simulink model "OscillatorAndLockin_Phase_or_Amp_FB_Mode"  (R2022b)
settings: Solver=VariableStepAuto  StartTime=0.0  StopTime=0.1  RelTol=1e-3
model workspace: external: MAT-File C:\Users\yoni\Documents\MATLAB\Examples\AFM\Dynamic Mode\WorkSpaceData.mat (data not in the file)
undefined symbols (not defined in the file or in its folder): ClockPeriod, D, I, N, P
libraries: simulink x7, slpidlib x2, simulink_extras x1
Description:
  | A model of the workings of "Phase or Amplitude feedback AFM (Atomic Force Microscopy)" aka "Tapping mode AFM"
  | This model contains:
  | a model of an AFM tip made of a tuning fork with tip-sample interaction force  i.e. a damped harmonic oscillator with external forces applied.
  | a model of a "Lock-in Amplifier",  with PLL mechanism that tracks the oscillator frequency.
  | 
  | The lock-in Amplifier does a "convolution" by multiplying its internal reference sin and cos signals with oscillator position signal, and summing each tick within a "time constant" period.
  | This splits the signal into symetric (cos) and antisymetric (sin) components. using euler
  | θ = tan-1 ( y / x )     r = √ ( x2 + y2 )
  | we can get esteemates for theta (phase) and r (amplitude)
  | lock-in then sythesize a sin signal amplitude of 1 and +90 degrees phase from the original position.
  | The oscillator is driven at it's own resonance frequency with a constant amplitude.
  | This is done by a controlled positive feedback loop, Autoresonance's force is amplified by a value designed to keep amplitude constant at setpoint.
  | (using a PID and the Lock-in's amplitude estimation)
  | 
  | The lock-in and PLL model uses the lock-in calculated phase and use that value to correct the lock-in's internal frequency
  | so it will match the external oscillator's frequency. (using another PID)
settings Model: PacingRate=1000  VariantFading=off  Creator=Yoni Cohen  LastModifiedBy=yoni
settings ConfigSet: Description=Current Conf
settings SolverCC: ZeroCrossAlgorithm=Adaptive  AlgebraicLoopSolver=LineSearch
settings DebuggingCC: UnconnectedInputMsg=warning  UnconnectedOutputMsg=warning  UnconnectedLineMsg=warning  UniqueDataStoreMsg=error  SFMachineParentedDataDiag=warning
settings HardwareCC: TargetBitPerPointer=64  TargetBitPerSizeT=64  TargetBitPerPtrDiffT=64  TargetLargestAtomicFloat=Float  TargetIntDivRoundTo=Zero  TargetEndianess=LittleEndian  TargetWordSize=64  TargetHWDeviceType=Intel->x86-64 (Windows64)  ProdEqTarget=off
settings ModelReferenceCC: EnableRefExpFcnMdlSchedulingChecks=on
settings SFSimCC: CustomCodeUndefinedFunction=UseInterfaceOnly

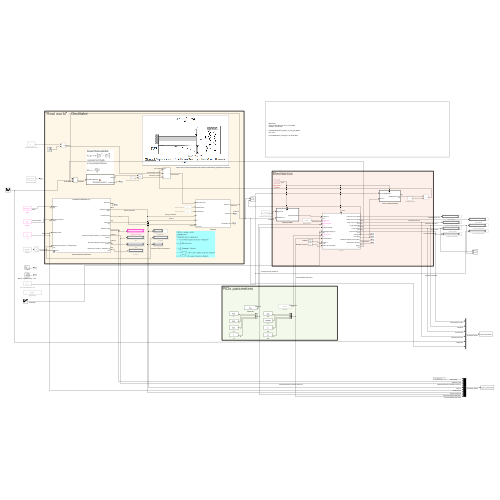
[thumbnail: Simulink's stored preview of the top-level diagram]
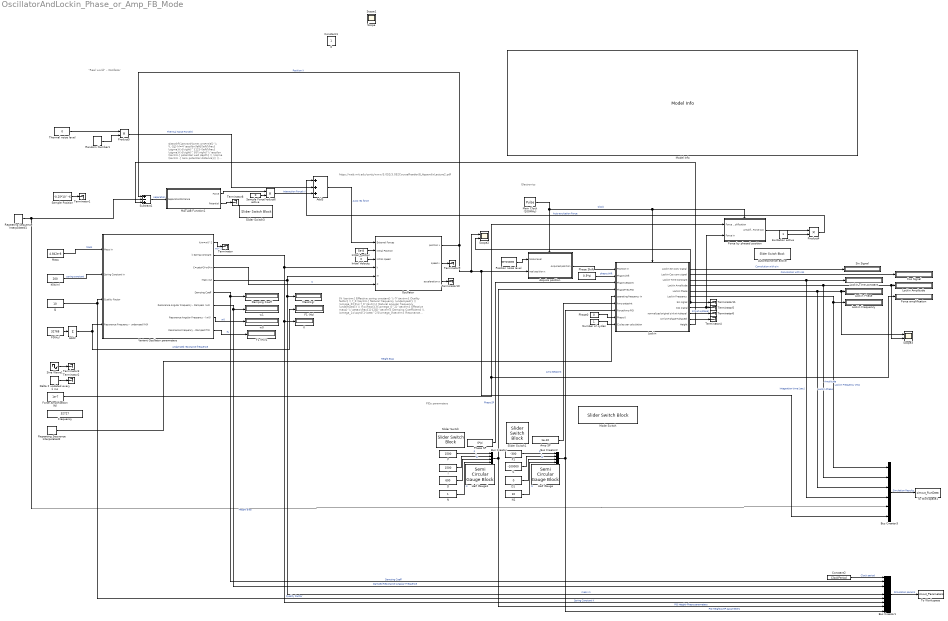
== system OscillatorAndLockin_Phase_or_Amp_FB_Mode ==
  note: $\textbf{Lennard-Jones potential} \\ V_{LJ}(r)=4 \epsilon\left[\left(\frac{ \sigma}{r}\right)^{12}-\left(\frac{ \sigma}{r}\right)^{6}\right] \\ \epsilon \textrm{ potential well depth} \\ \sigma \textrm { zero potential distance}\\ \\ F(r)=-\frac{\mathrm{d}V(r)}{\mathrm{d}r}$
  note: https://web.mit.edu/cortiz/www/3.052/3.052CourseReader/8_AppendixLecture2.pdf
  note: "Real world" - Oscillator
  note: Electronics
  note: PIDs parameters
  note: $k \textrm{ Effective spring constant} \\ Q \textrm{ Quality factor} \\ f_0 \textrm{ Natural frequency (undamped)} \\ \omega_0=2\pi f_0 \textrm{ Natural angular frequency (undamped)} \\ m=\frac{k}{\omega_0^2} \textrm{ Effective mass} \\ \zeta=\frac{1}{2Q} \textrm{ Damping Coefficient} \\ \omega_1=\sqrt{(1-\zeta^2)}\omega_0\textrm{ Resonance angular frequency (damped)} \\ f_1= \sqrt{(1-\zeta^2)}f_0\textrm{ Resonance frequency (damped)}$
  Acquire position : Subsystem
  Add2 : Sum  Inputs=+
  Add3 : Sum  Inputs=+++
  Amp SP : Constant  Value=1e-10  VectorParams1D=off  SampleTime=1e-5
  Autoresonance active : SliderSwitchBlock
      settings: Values={{'Off', 'On'}, [0 1]}
  Bus Creator : BusCreator  Inputs=P,I,D,N
  Bus Creator1 : BusCreator  Inputs=9
  Bus Creator2 : BusCreator  Inputs=P,I,D,N
  Bus Creator3 : BusCreator  Inputs=6
  Constant2 : Constant  Value=ClockPeriod
  Cos Signal : Display
  D : Constant  Value=600  SampleTime=1e-5
  D1 : Constant  Value=0  SampleTime=1e-5
  Damping Coeff : Display
  Delta F updated every 1 ms : RandomNumber  Variance=100  Seed=7546745  SampleTime=1e-3
  Excitation active : Constant  SampleTime=-1
  F0(Hz) : Constant  Value=32768
  F1 (Hz) : Display
  F1 (Hz)1 : Display
  Force Amplification (N) : Constant  Value=1e-7  SampleTime=-1
  Force amplification : Display
  Force by phased position : Subsystem  VariantControl=true
  Frequency : Constant  Value=32727  SampleTime=-1
  Half Gauge : SemiCircularGaugeBlock  LabelPosition=Bottom  ScaleMin=-10e-11  ScaleMax=10e-11
  Half Gauge1 : SemiCircularGaugeBlock  LabelPosition=Bottom  ScaleMin=-5e-4  ScaleMax=5e-4
  I : Constant  Value=1500  SampleTime=1e-5
  I1 : Constant  Value=-100000  VectorParams1D=off  SampleTime=1e-5
  Initial Position : Constant  Value=5e-8  VectorParams1D=off
  Initial Velocity : Constant  Value=0
  K : Display
  K(N/m) : Constant  Value=200
  Lockin : Subsystem
  Lockin Amplitude : Display
  Lockin Frequency : Display
  Lockin Phase : Display
  Lockin Time constant : Display
  MATLAB Function1 : MATLAB Function  TreatAsAtomicUnit=on
  Main Clock (100MHz) : DiscretePulseGenerator  PulseType=Time based  Period=ClockPeriod  PulseWidth=50
  Mass : Constant  Value=4.842e-8
  Mass(kg) : Display
      settings: Format=short_e
  Mode Switch : SliderSwitchBlock
      settings: Values={{'Amplitude FB', 'Phase FB'}, [0 1]}
  Model Info : simulink/Model-Wide Utilities/Model Info  Frame=on  DisplayStringWithTags=|  HorizontalTextAlignment=Left  LeftAlignmentValue=0.02
      | Model Info
      | Date Created %<Created>
      | Creator : %<Creator>
      | %<ModifiedComment>
      | %<ModelName> 
      | Ver. %<ModelVersion>
      | %<Description>
      | Last modification: %<LastModificationDate>
  N : Constant  SampleTime=1e-5
  N1 : Constant  Value=10  SampleTime=1e-5
  Number of cycles : Constant  OutDataTypeStr=uint16  SampleTime=-1
  Oscillator : Subsystem
  P : Constant  Value=1500  SampleTime=1e-5
  P1 : Constant  Value=-300  SampleTime=1e-5
  Phase SP : Constant  Value=0*pi  SampleTime=1e-5
  Phase Shift : Constant  Value=0.5*pi  VectorParams1D=off  SampleTime=-1
  Phase0 : Constant  Value=0  SampleTime=-1
  Position noise level : Constant  Value=0e-9/10000  VectorParams1D=off  SampleTime=-1
  Product4 : Product
  Product5 : Product
  Product6 : Product
  Q : Constant  Value=10
  Random Number1 : RandomNumber  Seed=754666  SampleTime=10^-8
  Repeating Sequence Interpolated1 : simulink/Sources/Repeating Sequence Interpolated  OutValues="[25e-10  0.6e-9 25e-10]"  TimeValues=[0 0.3 0.6]  LookUpMeth=Interpolation-Use End Values  tsamp=10^-5  OutMin=[]  OutMax=[]  OutDataTypeStr=double  OutputDataTypeScalingMode=double  OutDataType=fixdt(0,8)  OutScaling=2^-10
  Repeating Sequence Interpolated2 : simulink/Sources/Repeating Sequence Interpolated  OutValues="[32720  32800 32800]"  TimeValues=[0 0.1 0.11]  LookUpMeth=Interpolation-Use End Values  tsamp=10^-5  OutMin=[]  OutMax=[]  OutDataTypeStr=double  OutputDataTypeScalingMode=double  OutDataType=fixdt(0,8)  OutScaling=2^-10
  Sample Force active : Constant  Value=0  SampleTime=-1
  Sample Position : Constant  Value=-0.25*10^-6  SampleTime=-1
  Scope2 : Scope  NumInputPorts=2
  Scope3 : Scope  NumInputPorts=2
  Sin Signal : Display
  Sine Wave1 : Sin  Amplitude=20  Frequency=5000  Phase=0.0001  SampleTime=10e-6
  Slider Switch : SliderSwitchBlock
      settings: Values={{'Off', 'On'}, [0 1]}
  Slider Switch1 : SliderSwitchBlock
      settings: Values={{'Off', 'On'}, [0 1]}
  Slider Switch3 : SliderSwitchBlock
      settings: Values={{'Off', 'On'}, [0 1]}
  Subtract1 : Sum  Inputs=+-+  OutMin=[0]  RndMeth=Nearest
  Terminator{,1..6,8..11} (11 alike) : Terminator
  Thermal noise level : Constant  Value=0  VectorParams1D=off  SampleTime=-1
  To Workspace : ToWorkspace  VariableName=simout_Parameters  SaveFormat=Timeseries  SampleTime=1
  To Workspace1 : ToWorkspace  VariableName=simout_RunData  SaveFormat=Timeseries  SampleTime=1e-5
  Variant Oscillator parameters : Subsystem  Description=|  Variant=on  VariantControlMode=label  LabelModeActiveChoice=OscillatorTypeVar==0  PropagateVariantConditions=on
      | k  \textrm{ Effective spring constant.}
      | \\
      | Q  \textrm{ Quality factor.}
      | \\
      | f_0  \textrm{ Natural frequency undamped.}
      | \\
      | \omega_0=2\pi f_0 \textrm{ Natural angular frequency.}
      | \\
      | m=\frac{k}{\omega_0^2}  \textrm{ Effective mass.}
      | \\
      | \zeta=\frac{1}{2Q} \textrm{ Damping Coefficient.}
      | \\
      | \omega_1=\sqrt{(1-\zeta^2)}\omega_0\textrm{ Resonance angular frequency (damped)}
      | \\
      | f_1= \omega_1=\sqrt{(1-\zeta^2)}f_0\textrm{ Resonance frequency (damped)}
  w0 : Display
  w1 : Display
  0 : Constant  IOType=siggen
  Constant1 : Constant  IOType=siggen
  Scope : Scope
  Scope1 : Scope
  wires:
  Main Clock (100MHz)/1 -> Lockin/Trigger, Force by phased position/Trigger, Acquire position/Trigger  "Clock"
  Force by phased position/1(Amplified Force out) -> Product4/1
  Phase Shift/1 -> Lockin/2(Phase shift)  "phase shift"
  F0(Hz)/1 -> Add2/1
  Excitation active/1 -> Product4/2
  Random Number1/1 -> Product5/2
  Thermal noise level/1 -> Product5/1
  Sample Force active/1 -> Product6/2
  MATLAB Function1/1(Force) -> Product6/1
  Subtract1/1 -> MATLAB Function1/1(SeparationDistance)  "separation"
  K(N/m)/1 -> Variant Oscillator parameters/2(Spring Constant in)  "spring constant"
  Q/1 -> Variant Oscillator parameters/3(Quality Factor), Bus Creator1/6  "Quality Factor"
  Add2/1 -> Variant Oscillator parameters/4(Resonance Frequency - undamped (fr0)), F1 (Hz)/1  "undamped resonance frequence"
  Variant Oscillator parameters/6(Resonance Angular Frequency - Damped- (w1)) -> w1/1, Bus Creator1/3  "Damped Resonance Angular Frequence"
  Variant Oscillator parameters/4(Mass out) -> Mass(kg)/1, Bus Creator1/5, Oscillator/5(m)  "mass m"
  Variant Oscillator parameters/2(k Spring constant) -> Oscillator/4(k), K/1, Bus Creator1/7  "Spring Constant K"
  Variant Oscillator parameters/5(Damping Coeff) -> Damping Coeff/1, Bus Creator1/2  "Damping Coeff"
  Variant Oscillator parameters/7(Resonance Angular Frequency - (w0)) -> w0/1  "w0"
  Mass/1 -> Variant Oscillator parameters/1(Mass in)  "Mass"
  Variant Oscillator parameters/1(k/m=w0^2) -> Terminator/1  "w0^2"
  Lockin/2(Lockin Cos conv signal) -> Cos Signal/1  "Convolution with cos"
  Lockin/6(Lockin Frequency) -> Bus Creator3/1, Lockin Frequency/1  "Lockin Frequency [Hz]"
  Lockin/5(Lockin Phase) -> Bus Creator3/3, Scope3/1, Lockin Phase/1  "Lockin Phase"
  Lockin/3(Lockin Time Constant) -> Bus Creator3/4, Lockin Time constant/1  "Integration time [sec]"
  MATLAB Function1/2(Potential) -> Terminator8/1
  Lockin/4(Lockin Amplitude) -> Bus Creator3/2, Scope3/2, Lockin Amplitude/1  "Amplitude"
  Lockin/1(Lockin Sin conv signal) -> Sin Signal/1  "Convolution with sin"
  Acquire position/1(Acquired position) -> Lockin/1(Position in)
  Position noise level/1 -> Acquire position/1(Noise level)
  Phase SP/1 -> Lockin/3(Phase setpoint)  "Phase SP"
  I/1 -> Bus Creator/2  "I"
  D/1 -> Bus Creator/3  "D"
  P/1 -> Bus Creator/1  "P"
  N/1 -> Bus Creator/4  "N"
  Bus Creator/1 -> Lockin/4(Phase/Freq PID), Bus Creator1/8  "PID Height-Phase parameters"
  Product4/1 -> Add3/1  "Auto excitation Force"
  Phase0/1 -> Lockin/8(Phase 0)
  Delta F updated every 1 ms/1 -> Terminator2/1
  Lockin/8(Cos signal) -> Force by phased position/2(Force in), Terminator5/1
  Variant Oscillator parameters/8(Resonance Frequency - Damped (fr1)) -> F1 (Hz)1/1  "f1"
  Oscillator/1(" position x") -> Scope2/1, Bus Creator3/6, Acquire position/2(real position x), Subtract1/1  "Position X"
  Initial Position/1 -> Oscillator/2(Initial Position)
  Initial Velocity/1 -> Oscillator/3(Initial speed)
  Product6/1 -> Add3/3  "Interaction Force(x)"
  Variant Oscillator parameters/3(C=zeta*2*w0*m) -> Oscillator/6(C)  "C"
  Add3/1 -> Oscillator/1(External Forces)  "Auto res force"
  I1/1 -> Bus Creator2/2  "I"
  D1/1 -> Bus Creator2/3  "D"
  Bus Creator2/1 -> Bus Creator1/9, Lockin/7(Force/Amp PID)  "PID Height/AMP parameters"
  N1/1 -> Bus Creator2/4  "N"
  Sine Wave1/1 -> Terminator3/1
  Repeating Sequence Interpolated1/1 -> Subtract1/2, Bus Creator3/5  "Height Bias"
  P1/1 -> Bus Creator2/1  "P"
  Amp SP/1 -> Lockin/6(Amp setpoint)  "Amp Setpoint"
  Sample Position/1 -> Terminator1/1
  Bus Creator1/1 -> To Workspace/1  "Simulation params"
  Bus Creator3/1 -> To Workspace1/1  "Simulation Results"
  Constant2/1 -> Bus Creator1/1  "Clock period"
  Product5/1 -> Add3/2  "Thermal Noise Force(t)"
  Oscillator/2(speed v) -> Terminator9/1
  Oscillator/3(acceleration a) -> Terminator10/1
  Number of cycles/1 -> Lockin/9("Cycles per calculation ")
  Force Amplification (N)/1 -> Force amplification/1, Force by phased position/1(Force Amplification)
  Lockin/10(sin(wt+phase+phase0)) -> Terminator4/1
  Lockin/11(Height) -> Subtract1/3
  Lockin/7(Sin signal) -> Scope2/2, Terminator11/1
  Lockin/9(normalized original sin(wt+phase)) -> Terminator6/1  "sin(wt+phase)"
  Repeating Sequence Interpolated2/1 -> Lockin/5(operating frequency in)  "Height Bias"

== system OscillatorAndLockin_Phase_or_Amp_FB_Mode/Acquire position ==
  Noise level : Inport
  real position x : Inport  Port=2
  Trigger : TriggerPort  VariantControl=Variant  PortDimensions=1
  Add3 : Sum
  Product3 : Product
  Random Number : RandomNumber  Seed=7546767
  Acquired position : Outport  VectorParamsAs1DForOutWhenUnconnected=off
  wires:
  Product3/1 -> Add3/2  "Position acquisition error value"
  Random Number/1 -> Product3/2
  Noise level/1 -> Product3/1
  Add3/1 -> Acquired position/1  "Acquired position"
  real position x/1 -> Add3/1

== system OscillatorAndLockin_Phase_or_Amp_FB_Mode/Force by phased position ==
  Force Amplification : Inport
  Force in : Inport  Port=2
  Trigger : TriggerPort  VariantControl=Variant  PortDimensions=1
  Product3 : Product
  Amplified Force out : Outport  Unit=N  VectorParamsAs1DForOutWhenUnconnected=off
  wires:
  Product3/1 -> Amplified Force out/1
  Force in/1 -> Product3/2
  Force Amplification/1 -> Product3/1

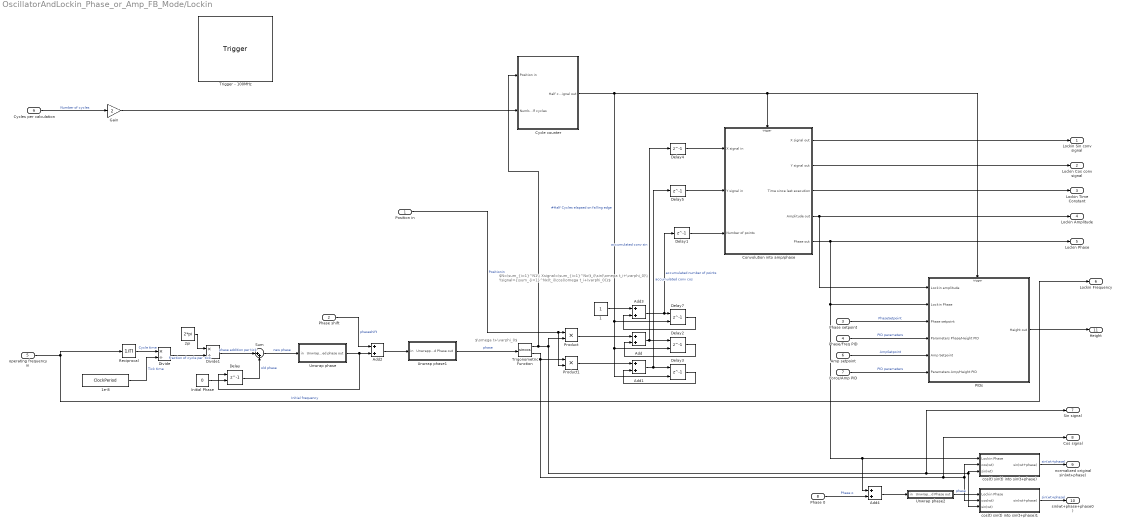
== system OscillatorAndLockin_Phase_or_Amp_FB_Mode/Lockin ==
  note: $N=\sum_{i=1}^N1\\ Xsignal=\sum_{i=1}^Nx(t_i)\sin(\omega t_i+\varphi_0)\\ Ysignal={\sum_{i=1}^Nx(t_i)\cos(\omega t_i+\varphi_0)}$
  note: $\omega t+\varphi_0$
  Position in : Inport  Unit=m
  Phase shift : Inport  Port=2  OutMin=[-2]  OutMax=[2]  Unit=rad
  Phase setpoint : Inport  Port=3  OutMin=[-2]  OutMax=[2]  Unit=rad
  Phase/Freq PID : Inport  Port=4
  operating frequency in : Inport  Port=5  Unit=Hz
  Amp setpoint : Inport  Port=6  Unit=m
  Force/Amp PID : Inport  Port=7
  Phase 0 : Inport  Port=8  Unit=rad
  "Cycles per calculation " : Inport  Port=9  OutDataTypeStr=uint16
  Trigger - 100MHz : TriggerPort  VariantControl=Variant  PortDimensions=1
  1 : Constant  OutDataTypeStr=Inherit: Inherit via back propagation
  1e-8 : Constant  Value=ClockPeriod  OutDataTypeStr=Inherit: Inherit via back propagation
  2pi : Constant  Value=2*pi  OutDataTypeStr=Inherit: Inherit via back propagation
  Add{,1..4} (5 alike) : Sum
  Convolution into amp/phase : Subsystem
  Cycle counter : Subsystem
  Delay : Delay  DelayLength=1  InitialConditionSource=Input port  InitialCondition=0
      settings: InputPortMap=u0,p4
  Delay1 : Delay  DelayLength=1  InitialCondition=0
  Delay2 : Delay  DelayLength=1  InitialCondition=0  ExternalReset=Falling
      settings: InputPortMap=u0,r5
  Delay3 : Delay  DelayLength=1  InitialCondition=0  ExternalReset=Falling
      settings: InputPortMap=u0,r5
  Delay4 : Delay  DelayLength=1  InitialCondition=0
  Delay5 : Delay  DelayLength=1  InitialCondition=0
  Delay7 : Delay  DelayLength=1  InitialCondition=0  ExternalReset=Falling
      settings: InputPortMap=u0,r5
  Divide : Product  Inputs=*/
  Divide1 : Product  Inputs=*/
  Gain : Gain  Gain=2  OutDataTypeStr=uint16
  Initial Phase : Constant  Value=0  OutDataTypeStr=Inherit: Inherit via back propagation
  PIDs : Subsystem
  Product : Product
  Product1 : Product
  Reciprocal : Product  Inputs=/
  Sum : Sum  Inputs=|++
  Trigonometric Function : Trigonometry  Operator=sincos  ApproximationMethod=CORDIC  NumberOfIterations=64
  Unwrap phase : Subsystem
  Unwrap phase1 : Subsystem
  Unwrap phase2 : Subsystem
  cos(t) sin(t) into sin(t+phase) : Subsystem
  cos(t) sin(t) into sin(t+phase)1 : Subsystem
  Lockin Sin conv signal : Outport  VectorParamsAs1DForOutWhenUnconnected=off
  Lockin Cos conv signal : Outport  Port=2  VectorParamsAs1DForOutWhenUnconnected=off
  Lockin Time Constant : Outport  Port=3  Unit=sec  VectorParamsAs1DForOutWhenUnconnected=off
  Lockin Amplitude : Outport  Port=4  Unit=m  VectorParamsAs1DForOutWhenUnconnected=off
  Lockin Phase : Outport  Port=5  Unit=rad  VectorParamsAs1DForOutWhenUnconnected=off
  Lockin Frequency : Outport  Port=6  Unit=Hz  InitialOutput=[32769]  VectorParamsAs1DForOutWhenUnconnected=off
  Sin signal : Outport  Port=7  VectorParamsAs1DForOutWhenUnconnected=off
  Cos signal : Outport  Port=8  VectorParamsAs1DForOutWhenUnconnected=off
  normalized original sin(wt+phase) : Outport  Port=9  VectorParamsAs1DForOutWhenUnconnected=off
  sin(wt+phase+phase0) : Outport  Port=10  VectorParamsAs1DForOutWhenUnconnected=off
  Height : Outport  Port=11  Unit=m  SourceOfInitialOutputValue=Input signal  InitialOutput=[32769]  VectorParamsAs1DForOutWhenUnconnected=off
  wires:
  Divide/1 -> Divide1/2  "fraction of cycle per  tick"
  2pi/1 -> Divide1/1
  Reciprocal/1 -> Divide/1  "Cycle time"
  Trigonometric Function/1 -> Cycle counter/1(Position in), Product/2, cos(t) sin(t) into sin(t+phase)/3(sin(wt)), cos(t) sin(t) into sin(t+phase)1/3(sin(wt)), Sin signal/1
  Trigonometric Function/2 -> Product1/1, Cos signal/1, cos(t) sin(t) into sin(t+phase)/2(cos(wt)), cos(t) sin(t) into sin(t+phase)1/2(cos(wt))
  1e-8/1 -> Divide/2  "Tick time"
  Position in/1 -> Product1/2, Product/1  "Positionin"
  Delay3/1 -> Add1/2
  Delay/1 -> Sum/2  "old phase"
  Delay2/1 -> Add/2
  Convolution into amp/phase/4(Amplitude out) -> Lockin Amplitude/1, PIDs/1(Lockin amplitude)
  Convolution into amp/phase/1(X signal out) -> Lockin Sin conv signal/1
  Convolution into amp/phase/2(Y signal out) -> Lockin Cos conv signal/1
  Add/1 -> Delay2/1, Delay4/1  "accumulated conv sin"
  Add1/1 -> Delay3/1, Delay5/1  "accumulated conv cos"
  Divide1/1 -> Sum/1  "phase addition per tick"
  Amp setpoint/1 -> PIDs/5(Amp Setpoint)  "AmpSetpoint"
  operating frequency in/1 -> Reciprocal/1, Lockin Frequency/1  "Initial frequency"
  Unwrap phase/1(Unwrapped phase out) -> Delay/1, Add2/2
  Sum/1 -> Unwrap phase/1(in)  "new phase"
  Add2/1 -> Unwrap phase1/1(in)
  Unwrap phase1/1(Unwrapped Phase out) -> Trigonometric Function/1  "phase"
  Gain/1 -> Cycle counter/2(Number of half cycles)
  Convolution into amp/phase/5(Phase out) -> cos(t) sin(t) into sin(t+phase)/1(Lockin Phase), Add4/1, PIDs/2(Lockin Phase), Lockin Phase/1
  Convolution into amp/phase/3(Time since last execution) -> Lockin Time Constant/1
  Product1/1 -> Add1/1
  Product/1 -> Add/1
  Delay5/1 -> Convolution into amp/phase/2(Y signal in)
  Delay4/1 -> Convolution into amp/phase/1(X signal in)
  Cycle counter/1(Half cycle counter signal out) -> Convolution into amp/phase/Trigger, PIDs/Trigger, Delay2/2, Delay3/2, Delay7/2  "#Half Cycles elapsed on falling edge"
  Add3/1 -> Delay1/1, Delay7/1  "accumulated number of points"
  Delay1/1 -> Convolution into amp/phase/3(Number of points)
  Phase shift/1 -> Add2/1  "phaseshift"
  Phase setpoint/1 -> PIDs/3(Phase setpoint)  "PhaseSetpoint"
  Initial Phase/1 -> Delay/2
  cos(t) sin(t) into sin(t+phase)/1(sin(wt+phase)) -> normalized original sin(wt+phase)/1  "sin(wt+phase)"
  Phase 0/1 -> Add4/2  "Phase o"
  Add4/1 -> Unwrap phase2/1(in)
  Unwrap phase2/1(Unwrapped Phase out) -> cos(t) sin(t) into sin(t+phase)1/1(Lockin Phase)  "phase"
  cos(t) sin(t) into sin(t+phase)1/1(sin(wt+phase)) -> sin(wt+phase+phase0)/1  "sin(wt+phase)"
  Force/Amp PID/1 -> PIDs/6(Parameters Amp/Height PID)  "PID parameters"
  1/1 -> Add3/1
  Delay7/1 -> Add3/2
  "Cycles per calculation "/1 -> Gain/1  "Number of cycles"
  Phase/Freq PID/1 -> PIDs/4(Parameters Phase/Height PID)  "PID parameters"
  PIDs/1(Height out) -> Height/1

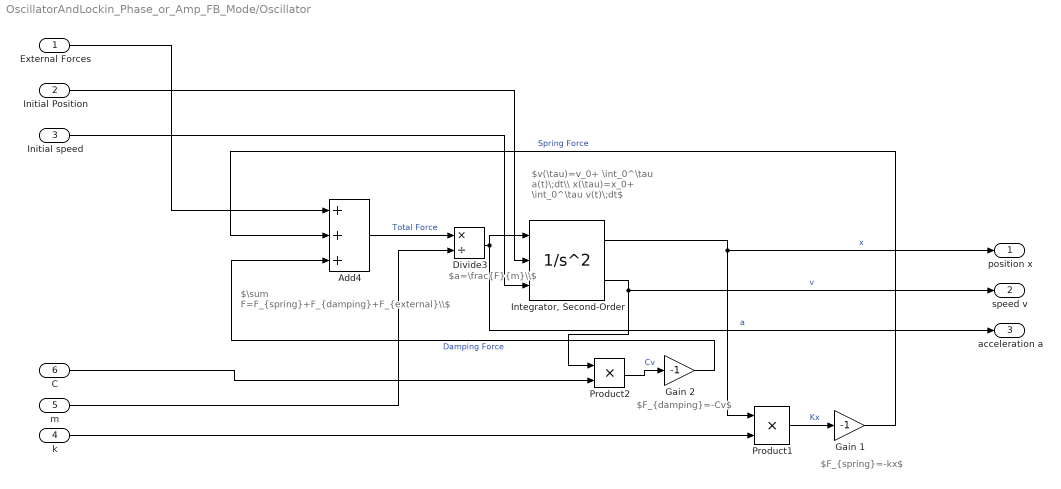
== system OscillatorAndLockin_Phase_or_Amp_FB_Mode/Oscillator ==
  note: $F_{spring}=-kx$
  note: $\sum F=F_{spring}+F_{damping}+F_{external}\\$
  note: $v(\tau)=v_0+ \int_0^\tau a(t)\;dt\\ x(\tau)=x_0+ \int_0^\tau v(t)\;dt$
  note: $a=\frac{F}{m}\\$
  note: $F_{damping}=-Cv$
  External Forces : Inport
  Initial Position : Inport  Port=2
  Initial speed : Inport  Port=3
  k : Inport  Port=4
  m : Inport  Port=5
  C : Inport  Port=6  Unit=N*sec/m
  Add4 : Sum  Inputs=+++
  Divide3 : Product  Inputs=*/
  Gain 1 : Gain  Gain=-1
  Gain 2 : Gain  Gain=-1
  "Integrator, Second-Order" : SecondOrderIntegrator  ICSourceX=external  LimitX=on  UpperLimitX=0.01  LowerLimitX=-0.01  StateNameX='x'  ICSourceDXDT=external  StateNameDXDT='v'
  Product1 : Product
  Product2 : Product
  " position x" : Outport
  speed v : Outport  Port=2
  acceleration a : Outport  Port=3
  wires:
  Divide3/1 -> "Integrator, Second-Order"/1, acceleration a/1  "a"
  Gain 2/1 -> Add4/3  "Damping Force"
  m/1 -> Divide3/2
  Product1/1 -> Gain 1/1  "Kx"
  C/1 -> Product2/2
  Initial speed/1 -> "Integrator, Second-Order"/3
  Add4/1 -> Divide3/1  "Total Force"
  External Forces/1 -> Add4/1
  Gain 1/1 -> Add4/2  "Spring Force"
  k/1 -> Product1/2
  "Integrator, Second-Order"/2 -> Product2/1, speed v/1  "v"
  Product2/1 -> Gain 2/1  "Cv"
  "Integrator, Second-Order"/1 -> " position x"/1, Product1/1  "x"
  Initial Position/1 -> "Integrator, Second-Order"/2

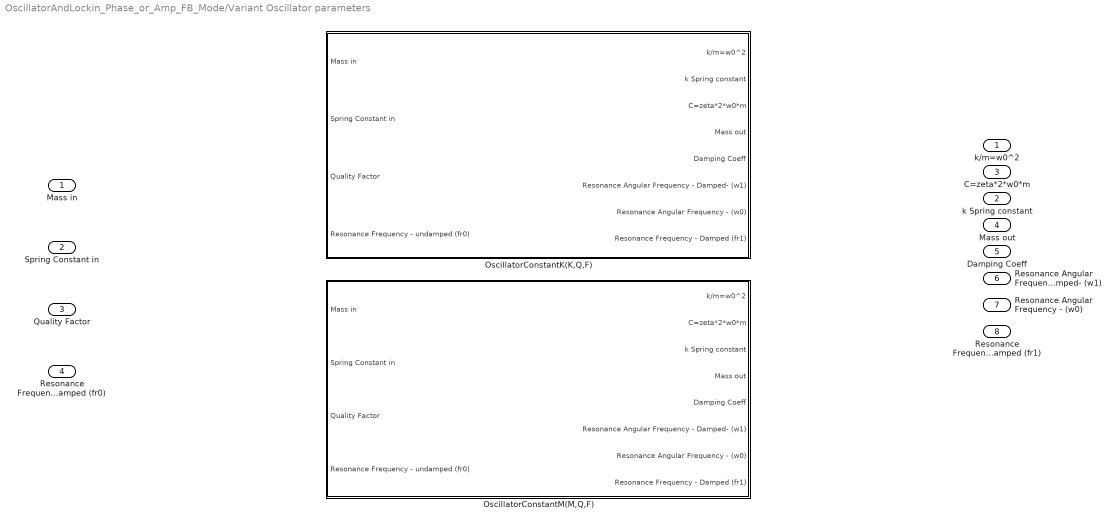
== system OscillatorAndLockin_Phase_or_Amp_FB_Mode/Variant Oscillator parameters ==
  Mass in : Inport  Unit=kg
  Spring Constant in : Inport  Port=2  Unit=N/m
  Quality Factor : Inport  Port=3
  Resonance Frequency - undamped (fr0) : Inport  Port=4  Unit=Hz
  OscillatorConstantK(K,Q,F) : Subsystem  VariantControl=OscillatorTypeVar==0
  OscillatorConstantM(M,Q,F) : Subsystem  VariantControl=OscillatorTypeVar==1
  k/m=w0^2 : Outport  VectorParamsAs1DForOutWhenUnconnected=off
  k Spring constant : Outport  Port=2  Unit=N/m  VectorParamsAs1DForOutWhenUnconnected=off
  C=zeta*2*w0*m : Outport  Port=3  VectorParamsAs1DForOutWhenUnconnected=off
  Mass out : Outport  Port=4  Unit=kg  VectorParamsAs1DForOutWhenUnconnected=off
  Damping Coeff : Outport  Port=5  VectorParamsAs1DForOutWhenUnconnected=off
  Resonance Angular Frequency - Damped- (w1) : Outport  Port=6  Unit=rad/sec  VectorParamsAs1DForOutWhenUnconnected=off
  Resonance Angular Frequency - (w0) : Outport  Port=7  Unit=rad/sec  VectorParamsAs1DForOutWhenUnconnected=off
  Resonance Frequency - Damped (fr1) : Outport  Port=8  Unit=Hz  VectorParamsAs1DForOutWhenUnconnected=off

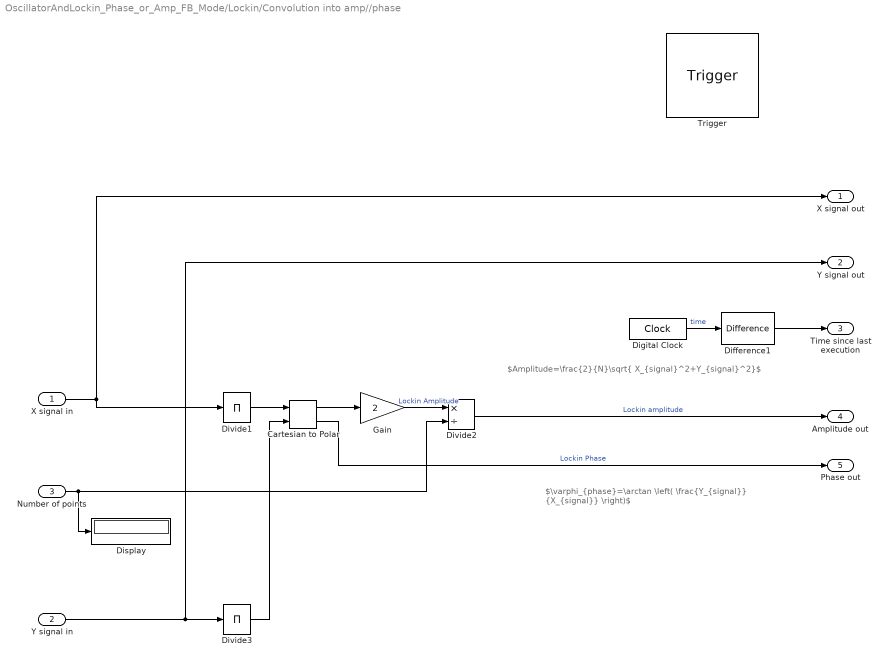
== system OscillatorAndLockin_Phase_or_Amp_FB_Mode/Lockin/Convolution into amp//phase ==
  note: $\varphi_{phase}=\arctan \left( \frac{Y_{signal}} {X_{signal}} \right)$
  note: $Amplitude=\frac{2}{N}\sqrt{ X_{signal}^2+Y_{signal}^2}$
  X signal in : Inport
  Y signal in : Inport  Port=2
  Number of points : Inport  Port=3
  Trigger : TriggerPort  TriggerType=falling  VariantControl=Variant  PortDimensions=1
  Cartesian to Polar : simulink_extras/Transformations/Cartesian to Polar
  Difference1 : simulink/Quick Insert/Discrete/Difference  ICPrevInput=0.0  OutMin=[]  OutMax=[]  OutDataType=fixdt(1, 16)  OutScaling=2^-10  DoSatur=off
  Digital Clock : DigitalClock  SampleTime=-1
  Display : Display
  Divide1 : Product  Inputs=*
  Divide2 : Product  Inputs=*/
  Divide3 : Product  Inputs=*
  Gain : Gain  Gain=2
  X signal out : Outport  VectorParamsAs1DForOutWhenUnconnected=off
  Y signal out : Outport  Port=2  VectorParamsAs1DForOutWhenUnconnected=off
  Time since last execution : Outport  Port=3  Unit=sec  VectorParamsAs1DForOutWhenUnconnected=off
  Amplitude out : Outport  Port=4  Unit=m  VectorParamsAs1DForOutWhenUnconnected=off
  Phase out : Outport  Port=5  Unit=rad  VectorParamsAs1DForOutWhenUnconnected=off
  wires:
  Cartesian to Polar/2 -> Phase out/1  "Lockin Phase"
  Digital Clock/1 -> Difference1/1  "time"
  Difference1/1 -> Time since last execution/1
  Gain/1 -> Divide2/1  "Lockin Amplitude"
  Number of points/1 -> Display/1, Divide2/2
  X signal in/1 -> Divide1/1, X signal out/1
  Y signal in/1 -> Y signal out/1, Divide3/1
  Cartesian to Polar/1 -> Gain/1
  Divide1/1 -> Cartesian to Polar/1
  Divide3/1 -> Cartesian to Polar/2
  Divide2/1 -> Amplitude out/1  "Lockin amplitude"

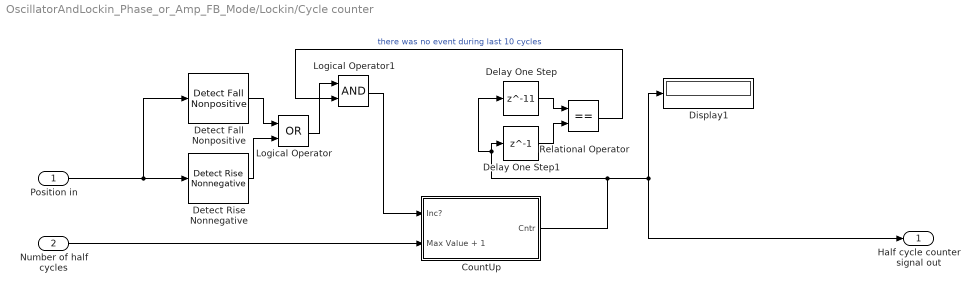
== system OscillatorAndLockin_Phase_or_Amp_FB_Mode/Lockin/Cycle counter ==
  Position in : Inport
  Number of half cycles : Inport  Port=2  OutDataTypeStr=uint16
  CountUp : Subsystem
  Delay One Step : Delay  DelayLength=11
  Delay One Step1 : Delay  DelayLength=1
  Detect Fall Nonpositive : simulink/Logic and Bit Operations/Detect Fall Nonpositive  vinit=0  OutDataTypeStr=boolean
  Detect Rise Nonnegative : simulink/Logic and Bit Operations/Detect Rise Nonnegative  vinit=0  OutDataTypeStr=boolean
  Display1 : Display
  Logical Operator : Logic  Operator=OR  AllPortsSameDT=off  OutDataTypeStr=boolean
  Logical Operator1 : Logic  AllPortsSameDT=off  OutDataTypeStr=boolean
  Relational Operator : RelationalOperator  Operator===  OutDataTypeStr=boolean  RndMeth=Simplest  InputSameDT=off
  Half cycle counter signal out : Outport  VectorParamsAs1DForOutWhenUnconnected=off
  wires:
  Detect Rise Nonnegative/1 -> Logical Operator/2
  Number of half cycles/1 -> CountUp/2(Max Value + 1)
  Position in/1 -> Detect Fall Nonpositive/1, Detect Rise Nonnegative/1
  Detect Fall Nonpositive/1 -> Logical Operator/1
  Logical Operator/1 -> Logical Operator1/1
  CountUp/1(Cntr) -> Delay One Step1/1, Delay One Step/1, Display1/1, Half cycle counter signal out/1
  Delay One Step/1 -> Relational Operator/1
  Delay One Step1/1 -> Relational Operator/2
  Relational Operator/1 -> Logical Operator1/2  "there was no event during last 10 cycles"
  Logical Operator1/1 -> CountUp/1(Inc?)

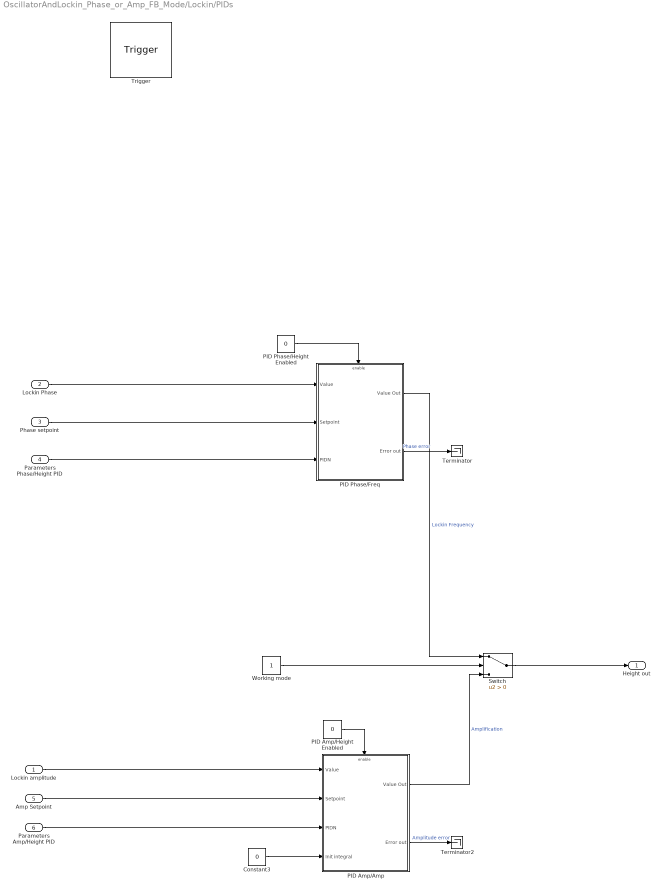
== system OscillatorAndLockin_Phase_or_Amp_FB_Mode/Lockin/PIDs ==
  Lockin amplitude : Inport
  Lockin Phase : Inport  Port=2
  Phase setpoint : Inport  Port=3
  Parameters Phase/Height PID : Inport  Port=4
  Amp Setpoint : Inport  Port=5
  Parameters Amp/Height PID : Inport  Port=6
  Trigger : TriggerPort  TriggerType=falling  VariantControl=Variant  PortDimensions=1
  Constant3 : Constant  Value=0
  PID Amp/Amp : Subsystem  TreatAsAtomicUnit=on
  PID Amp/Height Enabled : Constant  Value=0
  PID Phase/Freq : Subsystem  TreatAsAtomicUnit=on
  PID Phase/Height Enabled : Constant  Value=0
  Switch : Switch  Criteria=u2 > Threshold  SaturateOnIntegerOverflow=off  InputSameDT=off
  Terminator : Terminator
  Terminator2 : Terminator
  Working mode : Constant
  Height out : Outport  Unit=m  VectorParamsAs1DForOutWhenUnconnected=off
  wires:
  Phase setpoint/1 -> PID Phase/Freq/2(Setpoint)
  Amp Setpoint/1 -> PID Amp/Amp/2(Setpoint)
  Parameters Amp/Height PID/1 -> PID Amp/Amp/3(PIDN)
  PID Phase/Freq/1(Value Out) -> Switch/1  "Lockin Frequency"
  Lockin Phase/1 -> PID Phase/Freq/1(Value)
  PID Amp/Height Enabled/1 -> PID Amp/Amp/Enable
  Parameters Phase/Height PID/1 -> PID Phase/Freq/3(PIDN)
  Constant3/1 -> PID Amp/Amp/4(Init integral)
  PID Amp/Amp/1(Value Out) -> Switch/3  "Amplification"
  PID Phase/Freq/2(Error out) -> Terminator/1  "Phase error"
  PID Phase/Height Enabled/1 -> PID Phase/Freq/Enable
  PID Amp/Amp/2(Error out) -> Terminator2/1  "Amplitude error"
  Lockin amplitude/1 -> PID Amp/Amp/1(Value)
  Switch/1 -> Height out/1
  Working mode/1 -> Switch/2

== system OscillatorAndLockin_Phase_or_Amp_FB_Mode/Lockin/Unwrap phase ==
  in : Inport  Unit=rad
  2Pi : Constant  Value=2*pi  OutDataTypeStr=Inherit: Inherit via back propagation
  Relational Operator : RelationalOperator  Operator=<=  OutDataTypeStr=boolean  RndMeth=Simplest  InputSameDT=off
  Subtract : Sum  Inputs=+-
  Switch : Switch  Criteria=u2 > Threshold  SaturateOnIntegerOverflow=off  InputSameDT=off
  Unwrapped phase out : Outport  Unit=rad  VectorParamsAs1DForOutWhenUnconnected=off
  wires:
  Relational Operator/1 -> Switch/2
  in/1 -> Switch/1, Relational Operator/1, Subtract/1
  2Pi/1 -> Relational Operator/2, Subtract/2
  Subtract/1 -> Switch/3
  Switch/1 -> Unwrapped phase out/1

== system OscillatorAndLockin_Phase_or_Amp_FB_Mode/Lockin/Unwrap phase1 ==
  in : Inport
  Pi : Constant  Value=2*pi  OutDataTypeStr=Inherit: Inherit via back propagation
  Relational Operator : RelationalOperator  Operator=<=  OutDataTypeStr=boolean  RndMeth=Simplest  InputSameDT=off
  Subtract : Sum  Inputs=+-
  Switch : Switch  Criteria=u2 > Threshold  SaturateOnIntegerOverflow=off  InputSameDT=off
  Unwrapped Phase out : Outport  Unit=rad  VectorParamsAs1DForOutWhenUnconnected=off
  wires:
  Relational Operator/1 -> Switch/2
  in/1 -> Switch/1, Relational Operator/1, Subtract/1
  Switch/1 -> Unwrapped Phase out/1
  Pi/1 -> Relational Operator/2, Subtract/2
  Subtract/1 -> Switch/3

== system OscillatorAndLockin_Phase_or_Amp_FB_Mode/Lockin/Unwrap phase2 ==
  in : Inport
  Pi : Constant  Value=2*pi  OutDataTypeStr=Inherit: Inherit via back propagation
  Relational Operator : RelationalOperator  Operator=<=  OutDataTypeStr=boolean  RndMeth=Simplest  InputSameDT=off
  Subtract : Sum  Inputs=+-
  Switch : Switch  Criteria=u2 > Threshold  SaturateOnIntegerOverflow=off  InputSameDT=off
  Unwrapped Phase out : Outport  Unit=rad  VectorParamsAs1DForOutWhenUnconnected=off
  wires:
  Relational Operator/1 -> Switch/2
  in/1 -> Switch/1, Relational Operator/1, Subtract/1
  Switch/1 -> Unwrapped Phase out/1
  Pi/1 -> Relational Operator/2, Subtract/2
  Subtract/1 -> Switch/3

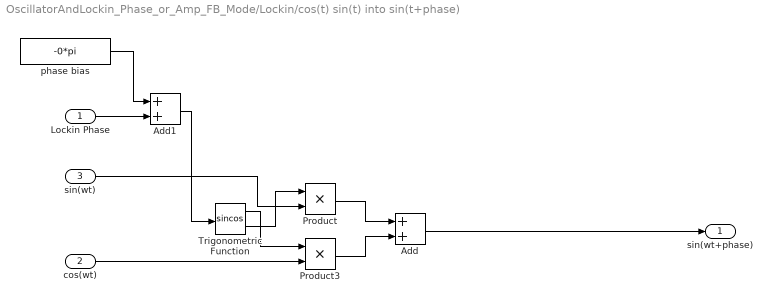
== system OscillatorAndLockin_Phase_or_Amp_FB_Mode/Lockin/cos(t) sin(t) into sin(t+phase) ==
  Lockin Phase : Inport  Unit=rad
  cos(wt) : Inport  Port=2
  sin(wt) : Inport  Port=3
  Add : Sum
  Add1 : Sum
  Product : Product
  Product3 : Product
  Trigonometric Function : Trigonometry  Operator=sincos  ApproximationMethod=CORDIC  NumberOfIterations=64
  phase bias : Constant  Value=-0*pi  SampleTime=-1
  sin(wt+phase) : Outport
  wires:
  Trigonometric Function/2 -> Product/1
  Trigonometric Function/1 -> Product3/1
  Product/1 -> Add/1
  sin(wt)/1 -> Product/2
  Product3/1 -> Add/2
  cos(wt)/1 -> Product3/2
  Add/1 -> sin(wt+phase)/1
  phase bias/1 -> Add1/1
  Lockin Phase/1 -> Add1/2
  Add1/1 -> Trigonometric Function/1

== system OscillatorAndLockin_Phase_or_Amp_FB_Mode/Lockin/cos(t) sin(t) into sin(t+phase)1 ==
  Lockin Phase : Inport  Unit=rad
  cos(wt) : Inport  Port=2
  sin(wt) : Inport  Port=3
  Add : Sum
  Add1 : Sum
  Product : Product
  Product3 : Product
  Trigonometric Function : Trigonometry  Operator=sincos  ApproximationMethod=CORDIC  NumberOfIterations=64
  phase bias : Constant  Value=-0*pi  SampleTime=-1
  sin(wt+phase) : Outport
  wires:
  Trigonometric Function/2 -> Product/1
  Trigonometric Function/1 -> Product3/1
  Product/1 -> Add/1
  sin(wt)/1 -> Product/2
  Product3/1 -> Add/2
  cos(wt)/1 -> Product3/2
  Add/1 -> sin(wt+phase)/1
  phase bias/1 -> Add1/1
  Lockin Phase/1 -> Add1/2
  Add1/1 -> Trigonometric Function/1

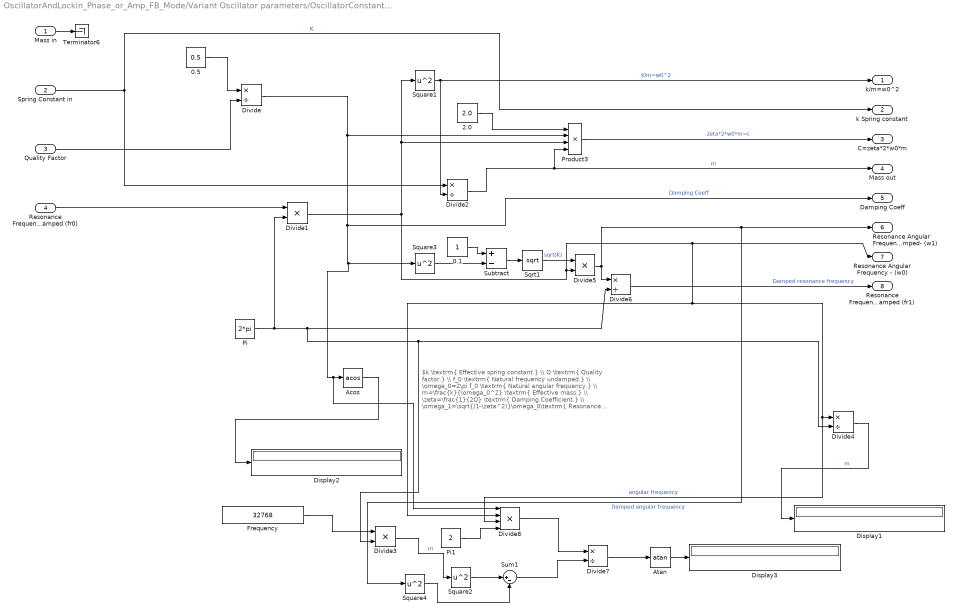
== system OscillatorAndLockin_Phase_or_Amp_FB_Mode/Variant Oscillator parameters/OscillatorConstantK(K,Q,F) ==
  note: $k \textrm{ Effective spring constant.} \\ Q \textrm{ Quality factor.} \\ f_0 \textrm{ Natural frequency undamped.} \\ \omega_0=2\pi f_0 \textrm{ Natural angular frequency.} \\ m=\frac{k}{\omega_0^2} \textrm{ Effective mass.} \\ \zeta=\frac{1}{2Q} \textrm{ Damping Coefficient.} \\ \omega_1=\sqrt{(1-\zeta^2)}\omega_0\textrm{ Resonance angular frequency (damped)} \\ f_1=\frac{\omega_1}{2\pi}=\sqrt{(1-\zeta^2)}f_0\textrm{ Resonance frequency (damped)}$
  Mass in : Inport  Unit=kg
  Spring Constant in : Inport  Port=2  Unit=N/m
  Quality Factor : Inport  Port=3
  Resonance Frequency - undamped (fr0) : Inport  Port=4  Unit=Hz
  0.1 : Constant
  0.5 : Constant  Value=0.5
  2.0 : Constant  Value=2.0
  Acos : Trigonometry  Operator=acos
  Atan : Trigonometry  Operator=atan
  Display1 : Display
  Display2 : Display
  Display3 : Display
  Divide{,2,4,6..7} (5 alike) : Product  Inputs=*/
  Divide1 : Product  Inputs=**
  Divide3 : Product  Inputs=**
  Divide5 : Product  Inputs=**
  Divide8 : Product  Inputs=****
  Frequency : Constant  Value=32768  SampleTime=-1
  Pi : Constant  Value=2*pi  OutDataTypeStr=Inherit: Inherit via back propagation
  Pi1 : Constant  Value=2  OutDataTypeStr=Inherit: Inherit via back propagation
  Product3 : Product  Inputs=4
  Sqrt1 : Sqrt
  Square{1..4} (4 alike) : Math  Operator=square  SignedPower=on
  Subtract : Sum  Inputs=+-
  Sum1 : Sum  Inputs=|+-
  Terminator6 : Terminator
  k/m=w0^2 : Outport  VectorParamsAs1DForOutWhenUnconnected=off
  k Spring constant : Outport  Port=2  Unit=N/m  VectorParamsAs1DForOutWhenUnconnected=off
  C=zeta*2*w0*m : Outport  Port=3  VectorParamsAs1DForOutWhenUnconnected=off
  Mass out : Outport  Port=4  Unit=kg  VectorParamsAs1DForOutWhenUnconnected=off
  Damping Coeff : Outport  Port=5  VectorParamsAs1DForOutWhenUnconnected=off
  Resonance Angular Frequency - Damped- (w1) : Outport  Port=6  Unit=rad/sec  VectorParamsAs1DForOutWhenUnconnected=off
  Resonance Angular Frequency - (w0) : Outport  Port=7  Unit=rad/sec  VectorParamsAs1DForOutWhenUnconnected=off
  Resonance Frequency - Damped (fr1) : Outport  Port=8  Unit=Hz  VectorParamsAs1DForOutWhenUnconnected=off
  wires:
  Divide1/1 -> Divide5/2, Divide8/3, Divide4/1, Divide8/2, Resonance Angular Frequency - (w0)/1, Square1/1, Product3/3  "angular frequency"
  Divide5/1 -> Divide6/1, Square4/1, Resonance Angular Frequency - Damped- (w1)/1  "Damped angular frequency"
  0.5/1 -> Divide/1
  Divide2/1 -> Product3/4, Mass out/1  "m"
  0.1/1 -> Subtract/1
  Divide/1 -> Divide8/1, Acos/1, Square3/1, Damping Coeff/1, Product3/2  "Damping Coeff"
  Square3/1 -> Subtract/2
  Sqrt1/1 -> Divide5/1  "sqrt(K)"
  Subtract/1 -> Sqrt1/1
  Square1/1 -> Divide2/2, k/m=w0^2/1  "k/m=w0^2"
  Pi/1 -> Divide1/2, Divide3/2, Divide4/2, Divide6/2
  2.0/1 -> Product3/1
  Resonance Frequency - undamped (fr0)/1 -> Divide1/1
  Quality Factor/1 -> Divide/2
  Product3/1 -> C=zeta*2*w0*m/1  "zeta*2*w0*m=c"
  Divide6/1 -> Resonance Frequency - Damped (fr1)/1  "Damped resonance frequency"
  Spring Constant in/1 -> Divide2/1, k Spring constant/1  "K"
  Mass in/1 -> Terminator6/1
  Divide4/1 -> Display1/1  "m"
  Acos/1 -> Display2/1
  Divide8/1 -> Divide7/1
  Sum1/1 -> Divide7/2
  Pi1/1 -> Divide8/4
  Square2/1 -> Sum1/1
  Divide7/1 -> Atan/1
  Atan/1 -> Display3/1
  Frequency/1 -> Divide3/1
  Divide3/1 -> Square2/1  "m"
  Square4/1 -> Sum1/2

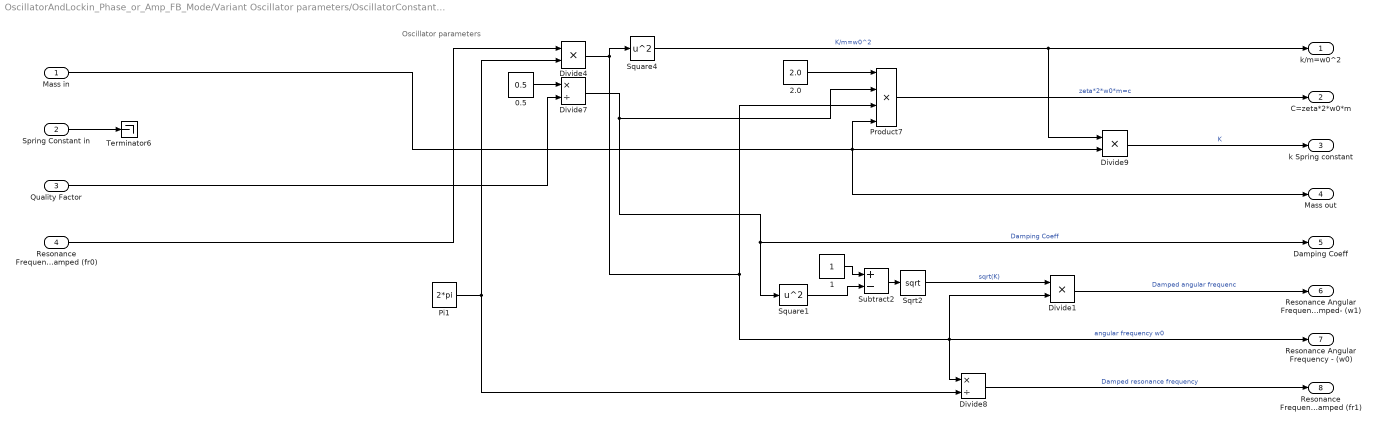
== system OscillatorAndLockin_Phase_or_Amp_FB_Mode/Variant Oscillator parameters/OscillatorConstantM(M,Q,F) ==
  note: Oscillator parameters
  Mass in : Inport  Unit=kg
  Spring Constant in : Inport  Port=2  Unit=N/m
  Quality Factor : Inport  Port=3
  Resonance Frequency - undamped (fr0) : Inport  Port=4  Unit=Hz
  0.5 : Constant  Value=0.5
  1 : Constant
  2.0 : Constant  Value=2.0
  Divide1 : Product  Inputs=**
  Divide4 : Product  Inputs=**
  Divide7 : Product  Inputs=*/
  Divide8 : Product  Inputs=*/
  Divide9 : Product  Inputs=**
  Pi1 : Constant  Value=2*pi  OutDataTypeStr=Inherit: Inherit via back propagation
  Product7 : Product  Inputs=4
  Sqrt2 : Sqrt
  Square1 : Math  Operator=square  SignedPower=on
  Square4 : Math  Operator=square  SignedPower=on
  Subtract2 : Sum  Inputs=+-
  Terminator6 : Terminator
  k/m=w0^2 : Outport  Unit=N/(kg*m)  VectorParamsAs1DForOutWhenUnconnected=off
  C=zeta*2*w0*m : Outport  Port=2  Unit=N*sec/kg/m  VectorParamsAs1DForOutWhenUnconnected=off
  k Spring constant : Outport  Port=3  Unit=N/m  VectorParamsAs1DForOutWhenUnconnected=off
  Mass out : Outport  Port=4  Unit=kg  VectorParamsAs1DForOutWhenUnconnected=off
  Damping Coeff : Outport  Port=5  VectorParamsAs1DForOutWhenUnconnected=off
  Resonance Angular Frequency - Damped- (w1) : Outport  Port=6  Unit=rad/sec  VectorParamsAs1DForOutWhenUnconnected=off
  Resonance Angular Frequency - (w0) : Outport  Port=7  Unit=rad/sec  VectorParamsAs1DForOutWhenUnconnected=off
  Resonance Frequency - Damped (fr1) : Outport  Port=8  Unit=Hz  VectorParamsAs1DForOutWhenUnconnected=off
  wires:
  Resonance Frequency - undamped (fr0)/1 -> Divide4/1
  Sqrt2/1 -> Divide1/1  "sqrt(K)"
  Square4/1 -> Divide9/1, k/m=w0^2/1  "K/m=w0^2"
  Pi1/1 -> Divide4/2, Divide8/2
  Divide7/1 -> Square1/1, Damping Coeff/1, Product7/2  "Damping Coeff"
  Divide4/1 -> Square4/1, Product7/3, Divide1/2, Divide8/1, Resonance Angular Frequency - (w0)/1  "angular frequency w0"
  Divide1/1 -> Resonance Angular Frequency - Damped- (w1)/1  "Damped angular frequenc"
  2.0/1 -> Product7/1
  Divide8/1 -> Resonance Frequency - Damped (fr1)/1  "Damped resonance frequency"
  Subtract2/1 -> Sqrt2/1
  Square1/1 -> Subtract2/2
  0.5/1 -> Divide7/1
  1/1 -> Subtract2/1
  Mass in/1 -> Mass out/1, Product7/4, Divide9/2
  Divide9/1 -> k Spring constant/1  "K"
  Product7/1 -> C=zeta*2*w0*m/1  "zeta*2*w0*m=c"
  Quality Factor/1 -> Divide7/2
  Spring Constant in/1 -> Terminator6/1

== system OscillatorAndLockin_Phase_or_Amp_FB_Mode/Lockin/Cycle counter/CountUp ==
  Inc? : Inport
  Max Value + 1 : Inport  Port=2
  2 : Constant  Value=0  OutDataTypeStr=uint16
  Delay One Step2 : Delay  DelayLength=1
  Increment Real World : simulink/Additional Math & Discrete/Additional Math: Increment - Decrement/Increment Real World
  Relational Operator1 : RelationalOperator  Operator=<  OutDataTypeStr=boolean  RndMeth=Simplest  InputSameDT=off
  Switch : Switch  Criteria=u2 ~= 0  SaturateOnIntegerOverflow=off  InputSameDT=off
  Switch1 : Switch  Criteria=u2 ~= 0  SaturateOnIntegerOverflow=off  InputSameDT=off
  Cntr : Outport  VectorParamsAs1DForOutWhenUnconnected=off
  wires:
  Switch/1 -> Delay One Step2/1
  Delay One Step2/1 -> Relational Operator1/1, Switch1/1
  Switch1/1 -> Cntr/1, Switch/3, Increment Real World/1
  Relational Operator1/1 -> Switch1/2
  2/1 -> Switch1/3
  Max Value + 1/1 -> Relational Operator1/2
  Increment Real World/1 -> Switch/1
  Inc?/1 -> Switch/2

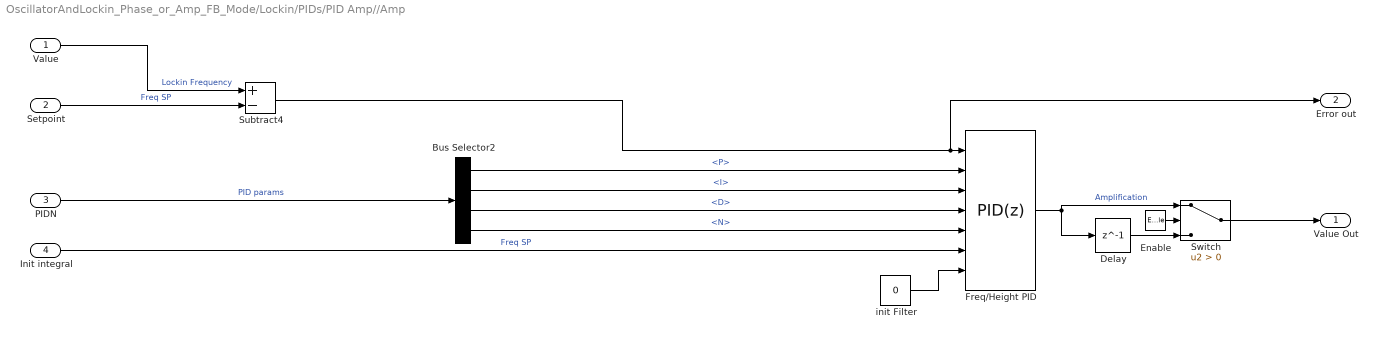
== system OscillatorAndLockin_Phase_or_Amp_FB_Mode/Lockin/PIDs/PID Amp//Amp ==
  Value : Inport
  Setpoint : Inport  Port=2
  PIDN : Inport  Port=3
  Init integral : Inport  Port=4
  Enable : EnablePort  ShowOutputPort=on
  Bus Selector2 : BusSelector  OutputSignals=P,I,D,N
  Delay : Delay  DelayLength=1  InitialCondition=0
  Freq/Height PID : slpidlib/PID Controller  Controller=PID  Form=Parallel  TimeDomain=Discrete-time  UseExternalTs=off  SampleTime=-1  IntegratorMethod=Forward Euler  FilterMethod=Forward Euler  ControllerParametersSource=external  P=20  I=100  UseKiTs=off  D=1400  N=1  UseFilter=on  TunerSelectOption=Transfer Function Based (PID Tuner App)  InitialConditionSource=external  InitialConditionForIntegrator=0  InitialConditionForFilter=0  DifferentiatorICPrevScaledInput=0  ExternalReset=none  TrackingMode=off  Kt=1  LimitOutput=off  SatLimitsSource=internal  UpperSaturationLimit=inf  LowerSaturationLimit=-inf  LinearizeAsGain=off  AntiWindupMode=none  Kb=1  LimitIntegrator=off  UpperIntegratorSaturationLimit=inf  LowerIntegratorSaturationLimit=-inf  RndMeth=Round  POutMin=[]  POutMax=[]  IOutMin=[]  IOutMax=[]  DOutMin=[]  DOutMax=[]  NOutMin=[]  NOutMax=[]  SumOutMin=[]  SumOutMax=[]  SaturationOutMin=[]  SaturationOutMax=[]  PParamMin=[]  PParamMax=[]  IParamMin=[]  IParamMax=[]  DParamMin=[]  DParamMax=[]  NParamMin=[]  NParamMax=[]  KbParamMin=[]  KbParamMax=[]  KtParamMin=[]  KtParamMax=[]  KbOutMin=[]  KbOutMax=[]  KtOutMin=[]  KtOutMax=[]  IntegratorOutMin=[]  IntegratorOutMax=[]  FilterOutMin=[]  FilterOutMax=[]  SumI1OutMin=[]  SumI1OutMax=[]  SumI2OutMin=[]  SumI2OutMax=[]  SumI3OutMin=[]  SumI3OutMax=[]  SumI4OutMin=[]  SumI4OutMax=[]  SumDOutMin=[]  SumDOutMax=[]  DifferentiatorOutMin=[]  DifferentiatorOutMax=[]  FilterDiffOutCoefMin=[]  FilterDiffOutCoefMax=[]  ReciprocalOutMin=[]  ReciprocalOutMax=[]  SumDenOutMin=[]  SumDenOutMax=[]  SumNumOutMin=[]  SumNumOutMax=[]  DivideOutMin=[]  DivideOutMax=[]  UdiffTsProdOutMin=[]  UdiffTsProdOutMax=[]  NTsProdOutMin=[]  NTsProdOutMax=[]  UintegralTsProdOutMin=[]  UintegralTsProdOutMax=[]  UngainTsProdOutMin=[]  UngainTsProdOutMax=[]  ClampingZeroOutDataTypeStr=Inherit: Inherit via back propagation  ClampingZeroOutMin=[]  ClampingZeroOutMax=[]  FilterDenConstantOutDataTypeStr=Inherit: Inherit via back propagation  FilterDenConstantOutMin=[]  FilterDenConstantOutMax=[]  PCopyOutDataTypeStr=Inherit: Inherit via back propagation  PCopyOutMin=[]  PCopyOutMax=[]  NCopyOutDataTypeStr=Inherit: Inherit via back propagation  NCopyOutMin=[]  NCopyOutMax=[]  IntegratorContinuousStateAttributes=''  IntegratorStateMustResolveToSignalObject=off  IntegratorRTWStateStorageClass=Auto  FilterContinuousStateAttributes=''  FilterStateMustResolveToSignalObject=off  FilterRTWStateStorageClass=Auto  ParallelPVariant=ExternalParameters  IdealPVariant=Disabled  IVariant=ExternalParameters  DVariant=ExternalParameters  IntegratorVariant=Discrete  SatVariant=Disabled  AWVariant=Passthrough  PCopyVariant=Disabled  TRVariant=Disabled  FdbkBlocksVariant=Forward  IdealPFdbkVariant=Disabled  SatFdbkVariant=Disabled  DerivativeFilterVariant=ForwardEulerFilter  NVariant=ExternalParameters  NCopyVariant=Disabled  FilterICVariant=ExternalICs  IntegratorICVariant=ExternalICs  ExternalResetVariant=Disabled  TRSumVariant=Passthrough  SumFdbkVariant=Disabled  SumVariant=Sum_PID  TsampFilterVariant=InternalTs  TsampNgainVariant=Passthrough  TsampIntegralVariant=Passthrough  ExternalSaturationOutDataTypeStr=Inherit: Same as second input
  Subtract4 : Sum  Inputs=+-
  Switch : Switch  Criteria=u2 > Threshold  SaturateOnIntegerOverflow=off  InputSameDT=off
  init Filter : Constant  Value=0
  Value Out : Outport
  Error out : Outport  Port=2
  wires:
  Subtract4/1 -> Error out/1, Freq/Height PID/1
  Setpoint/1 -> Subtract4/2  "Freq SP"
  Bus Selector2/2 -> Freq/Height PID/3  "<I>"
  Bus Selector2/3 -> Freq/Height PID/4  "<D>"
  PIDN/1 -> Bus Selector2/1  "PID params"
  Value/1 -> Subtract4/1  "Lockin Frequency"
  Bus Selector2/4 -> Freq/Height PID/5  "<N>"
  Bus Selector2/1 -> Freq/Height PID/2  "<P>"
  Freq/Height PID/1 -> Switch/1, Delay/1  "Amplification"
  Delay/1 -> Switch/3
  Enable/1 -> Switch/2
  Switch/1 -> Value Out/1
  Init integral/1 -> Freq/Height PID/6  "Freq SP"
  init Filter/1 -> Freq/Height PID/7

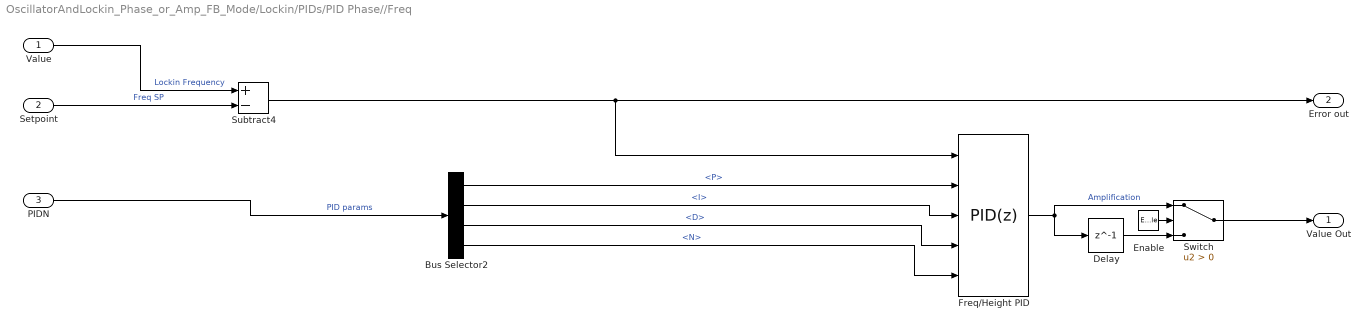
== system OscillatorAndLockin_Phase_or_Amp_FB_Mode/Lockin/PIDs/PID Phase//Freq ==
  Value : Inport
  Setpoint : Inport  Port=2
  PIDN : Inport  Port=3
  Enable : EnablePort  ShowOutputPort=on
  Bus Selector2 : BusSelector  OutputSignals=P,I,D,N
  Delay : Delay  DelayLength=1  InitialCondition=0
  Freq/Height PID : slpidlib/PID Controller  Controller=PID  Form=Parallel  TimeDomain=Discrete-time  UseExternalTs=off  SampleTime=-1  IntegratorMethod=Forward Euler  FilterMethod=Forward Euler  ControllerParametersSource=external  P=20  I=100  UseKiTs=off  D=1400  N=1  UseFilter=on  TunerSelectOption=Transfer Function Based (PID Tuner App)  InitialConditionSource=internal  InitialConditionForIntegrator=0  InitialConditionForFilter=0  DifferentiatorICPrevScaledInput=0  ExternalReset=none  TrackingMode=off  Kt=1  LimitOutput=off  SatLimitsSource=internal  UpperSaturationLimit=inf  LowerSaturationLimit=-inf  LinearizeAsGain=off  AntiWindupMode=none  Kb=1  LimitIntegrator=off  UpperIntegratorSaturationLimit=inf  LowerIntegratorSaturationLimit=-inf  RndMeth=Round  POutMin=[]  POutMax=[]  IOutMin=[]  IOutMax=[]  DOutMin=[]  DOutMax=[]  NOutMin=[]  NOutMax=[]  SumOutMin=[]  SumOutMax=[]  SaturationOutMin=[]  SaturationOutMax=[]  PParamMin=[]  PParamMax=[]  IParamMin=[]  IParamMax=[]  DParamMin=[]  DParamMax=[]  NParamMin=[]  NParamMax=[]  KbParamMin=[]  KbParamMax=[]  KtParamMin=[]  KtParamMax=[]  KbOutMin=[]  KbOutMax=[]  KtOutMin=[]  KtOutMax=[]  IntegratorOutMin=[]  IntegratorOutMax=[]  FilterOutMin=[]  FilterOutMax=[]  SumI1OutMin=[]  SumI1OutMax=[]  SumI2OutMin=[]  SumI2OutMax=[]  SumI3OutMin=[]  SumI3OutMax=[]  SumI4OutMin=[]  SumI4OutMax=[]  SumDOutMin=[]  SumDOutMax=[]  DifferentiatorOutMin=[]  DifferentiatorOutMax=[]  FilterDiffOutCoefMin=[]  FilterDiffOutCoefMax=[]  ReciprocalOutMin=[]  ReciprocalOutMax=[]  SumDenOutMin=[]  SumDenOutMax=[]  SumNumOutMin=[]  SumNumOutMax=[]  DivideOutMin=[]  DivideOutMax=[]  UdiffTsProdOutMin=[]  UdiffTsProdOutMax=[]  NTsProdOutMin=[]  NTsProdOutMax=[]  UintegralTsProdOutMin=[]  UintegralTsProdOutMax=[]  UngainTsProdOutMin=[]  UngainTsProdOutMax=[]  ClampingZeroOutDataTypeStr=Inherit: Inherit via back propagation  ClampingZeroOutMin=[]  ClampingZeroOutMax=[]  FilterDenConstantOutDataTypeStr=Inherit: Inherit via back propagation  FilterDenConstantOutMin=[]  FilterDenConstantOutMax=[]  PCopyOutDataTypeStr=Inherit: Inherit via back propagation  PCopyOutMin=[]  PCopyOutMax=[]  NCopyOutDataTypeStr=Inherit: Inherit via back propagation  NCopyOutMin=[]  NCopyOutMax=[]  IntegratorContinuousStateAttributes=''  IntegratorStateMustResolveToSignalObject=off  IntegratorRTWStateStorageClass=Auto  FilterContinuousStateAttributes=''  FilterStateMustResolveToSignalObject=off  FilterRTWStateStorageClass=Auto  ParallelPVariant=ExternalParameters  IdealPVariant=Disabled  IVariant=ExternalParameters  DVariant=ExternalParameters  IntegratorVariant=Discrete  SatVariant=Disabled  AWVariant=Passthrough  PCopyVariant=Disabled  TRVariant=Disabled  FdbkBlocksVariant=Forward  IdealPFdbkVariant=Disabled  SatFdbkVariant=Disabled  DerivativeFilterVariant=ForwardEulerFilter  NVariant=ExternalParameters  NCopyVariant=Disabled  FilterICVariant=InternalICsFilter  IntegratorICVariant=InternalICs  ExternalResetVariant=Disabled  TRSumVariant=Passthrough  SumFdbkVariant=Disabled  SumVariant=Sum_PID  TsampFilterVariant=InternalTs  TsampNgainVariant=Passthrough  TsampIntegralVariant=Passthrough  ExternalSaturationOutDataTypeStr=Inherit: Same as second input
  Subtract4 : Sum  Inputs=+-
  Switch : Switch  Criteria=u2 > Threshold  SaturateOnIntegerOverflow=off  InputSameDT=off
  Value Out : Outport
  Error out : Outport  Port=2
  wires:
  Subtract4/1 -> Freq/Height PID/1, Error out/1
  Setpoint/1 -> Subtract4/2  "Freq SP"
  Bus Selector2/2 -> Freq/Height PID/3  "<I>"
  Bus Selector2/3 -> Freq/Height PID/4  "<D>"
  PIDN/1 -> Bus Selector2/1  "PID params"
  Value/1 -> Subtract4/1  "Lockin Frequency"
  Bus Selector2/4 -> Freq/Height PID/5  "<N>"
  Bus Selector2/1 -> Freq/Height PID/2  "<P>"
  Freq/Height PID/1 -> Switch/1, Delay/1  "Amplification"
  Delay/1 -> Switch/3
  Enable/1 -> Switch/2
  Switch/1 -> Value Out/1

== matlab function OscillatorAndLockin_Phase_or_Amp_FB_Mode/MATLAB Function1 ==
  data: SeparationDistance input; Force output; Potential output
%% Calculates the interaction Force and Potential as a function of seperation distance
function [Force,Potential] = TipSampleInteraction(SeparationDistance)
[Potential,Force] = sampledistanceLJ(SeparationDistance);
